simulink model "Demo_vehicle"  (Simulink 7.0)
settings: Solver=ode1  StartTime=0.0  StopTime=inf  FixedStep=0.001  RelTol=1e-3
values from neighbouring files (symbols this model uses):
  map = round(map)    [Demo_init.m]
libraries: quarc_library x2, vrlib x1
settings Model: Creator=colinlea  LastModifiedBy=colinlea  SimulationMode=external  ExtModeTrigDuration=10000
settings SolverCC: PositivePriorityOrder=on
settings RTWCC: SystemTargetFile=quarc_windows.tlc  TemplateMakefile=quarc_default_tmf  Description=QuaRC Win32 Target  ProcessScript=quarc_windows_make_rtw_hook
settings STFCustomTargetCC: TargetPreCompLibLocation=C:\DOCUME~1\ALLUSE~1\APPLIC~1\QuaRC\lib\2007b\windows\release  GenFloatMathFcnCalls=ANSI_C  SystemTargetFile=quarc_windows.tlc
settings GRTTargetCC: TargetPreCompLibLocation=C:\DOCUME~1\ALLUSE~1\APPLIC~1\QuaRC\lib\2007b\windows\release  CompOptLevelCompliant=off  MatFileLogging=off  ExtMode=on  ExtModeMexFile=quarc_comm

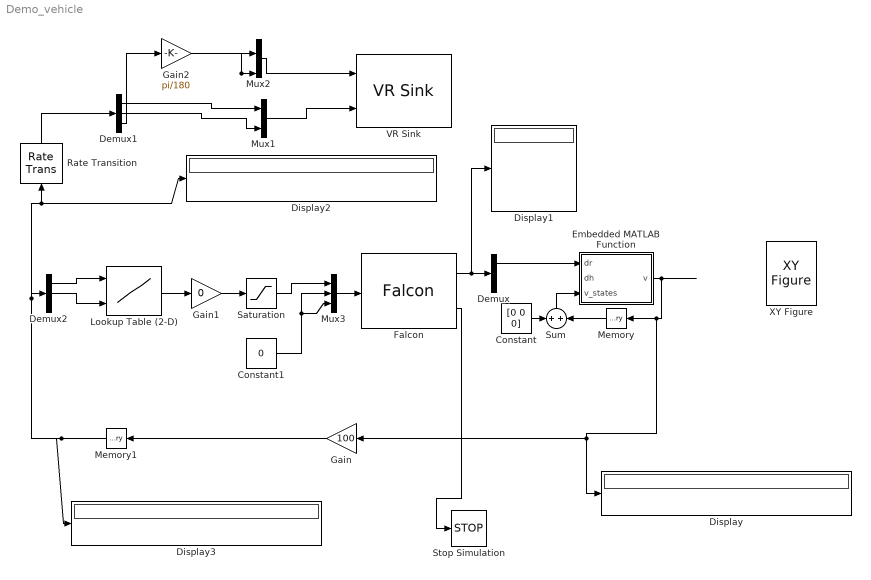
== system Demo_vehicle ==
  Constant : Constant  Value=[0 0 0]  OutDataType=sfix(16)  OutScaling=2^0
  Constant1 : Constant  Value=0  OutDataType=sfix(16)  OutScaling=2^0
  Demux : Demux  Outputs=3
  Demux1 : Demux  Outputs=3
  Demux2 : Demux  Outputs=3
  Display{,1..3} (4 alike) : Display
  Embedded MATLAB Function : Stateflow chart
  Falcon : quarc_library/Devices/Third-Party/Novint/Falcon  sample_time=qc_get_step_size  show_calibrate=off
  Gain : Gain  Orientation=left  Gain=100  ParameterDataType=sfix(16)  ParameterScaling=2^0  OutDataType=sfix(16)  OutScaling=2^0
  Gain1 : Gain  Gain=0  ParameterDataType=sfix(16)  ParameterScaling=2^0  OutDataType=sfix(16)  OutScaling=2^0
  Gain2 : Gain  Gain=pi/180  ParameterDataType=sfix(16)  ParameterScaling=2^0  OutDataType=sfix(16)  OutScaling=2^0
  Lookup Table (2-D) : Lookup2D  RowIndex=[1:100]  ColumnIndex=[1:100]  Table=map  OutDataType=sfix(16)  OutScaling=2^0
  Memory : Memory  Orientation=left
  Memory1 : Memory  Orientation=left
  Mux1 : Mux  Inputs=3
  Mux2 : Mux
  Mux3 : Mux  Inputs=3
  Rate Transition : RateTransition  Orientation=up  OutPortSampleTime=.1
  Saturation : Saturate  UpperLimit=5  LowerLimit=-5  OutDataType=sfix(16)  OutScaling=2^0
  Stop Simulation : Stop
  Sum : Sum  Orientation=up  Inputs=+|+  OutDataType=sfix(16)  OutScaling=2^0
  VR Sink : vrlib/VR Sink  SampleTime=0.1  ViewEnable=on  RemoteChange=off  RemoteView=on  FieldsWritten=Vehicle.rotation.4.1.double#Vehicle.translation.3.1.double  WorldFileName=demo_basic.wrl  AutoView=off  VideoDimensions=[]  FigureProperties="{'Position', 'Name', 'Viewpoint', 'CameraBound', 'CameraDirection', 'CameraPosition', 'CameraUpVector', 'ZoomFactor', 'Antialiasing', 'Headlight', 'Lighting', 'NavPanel', 'StatusBar', 'ToolBar', 'Textures', 'Transparency', 'Wireframe', 'NavZones', 'NavMode', 'NavSpeed', 'Record2DCompressMethod', 'Record2DCompressQuality', 'Record2D', 'Record2DFileName', 'Record2DFPS'; [5.0000000000000000e+000  9.2000000000000000e+001  5.7600000000000000e+002  3.8000000000000000e+002], '', '', 'on', [2.1160629078551965e-001 -3.4517254280434406e-001 -9.1437338838900839e-001], [1.2830017176593078e+000  1.1093262450780815e+001  5.7975808047642531e+001], [-5.6703177561002682e-002  9.2964749193693252e-001 -3.6406083336424244e-001], [1.0000000000000000e+000], 'off', 'on', 'on', 'halfbar', 'off', 'on', 'on', 'on', 'off', 'off', 'fly', 'normal', 'auto', [7.5000000000000000e+001], 'off', '%f_anim_%n.avi', [1.5000000000000000e+001]}"
  XY Figure : quarc_library/Sinks/Figures/XY Figure  figure_mode=Use figure window  figure_tag=figure1  axes_tag=axes1  minimum_x=-1  maximum_x=1  minimum_y=-1  maximum_y=1  trace_mode=Erase old trace  buffer_size=1000  update_rate=100  sample_time=-1
  wires:
  Falcon/1 -> Demux/1, Display1/1
  Embedded MATLAB Function/1(v) -> Memory/1, Display/1, Gain/1
  ? -> XY Figure/1
  ? -> XY Figure/2
  Constant/1 -> Sum/1
  Memory/1 -> Sum/2
  Sum/1 -> Embedded MATLAB Function/3(v_states)
  Demux/1 -> Embedded MATLAB Function/1(dr)
  Demux2/1 -> Lookup Table (2-D)/1
  Demux2/2 -> Lookup Table (2-D)/2
  Gain/1 -> Memory1/1
  Lookup Table (2-D)/1 -> Gain1/1
  Gain1/1 -> Saturation/1
  Saturation/1 -> Mux3/1
  Constant1/1 -> Mux3/2, Mux3/3
  Mux3/1 -> Falcon/1
  Memory1/1 -> Demux2/1, Display2/1, Rate Transition/1, Display3/1
  Demux1/1 -> Mux1/1
  Demux1/2 -> Mux1/3
  Demux1/3 -> Gain2/1
  Mux2/1 -> VR Sink/1
  Mux1/1 -> VR Sink/2
  Falcon/2 -> Stop Simulation/1
  Rate Transition/1 -> Demux1/1
  Gain2/1 -> Mux2/2, Mux2/4

== matlab function Embedded MATLAB Function ==
  data: dr input inherited; dh input inherited; v output inherited; v_states input inherited
function v = fcn( dr, dh, v_states)
% This block supports the Embedded MATLAB subset.
% See the help menu for details. 

v = [v_states(1)+dr*cos(v_states(3))*.01, v_states(2)+dr*sin(v_states(3))*.01, v_states(3)-.1*dh];
